simulink model "L400_airframe"  (R2024b)
settings: Solver=FixedStepAuto  StartTime=0  StopTime=20  FixedStep=5/1000  RelTol=1e-3
model workspace (MAT data in the model file):
  Sig : Simulink.Signal (value not decoded)
  Sig1 : Simulink.Signal (value not decoded)
  Sig2 : Simulink.Signal (value not decoded)
  Sig3 : Simulink.Signal (value not decoded)
  Sig4 : Simulink.Signal (value not decoded)
  Sig5 : Simulink.Signal (value not decoded)
  Sig6 : Simulink.Signal (value not decoded)
undefined symbols (not defined in the file or in its folder): convertTo, datetime, db, Earth, F, lambda, Light, MIL, WGS84, WMM2020
libraries: aerolibconvert2 x18, aerolibasang x5, aerolibtransform2 x3, aerolibwind2 x3, aerolibactuator x2, matrix_library x2, shared6dof x1, aerolibatmos2 x1, aerolibgravity2 x1
(part 3 of 4)

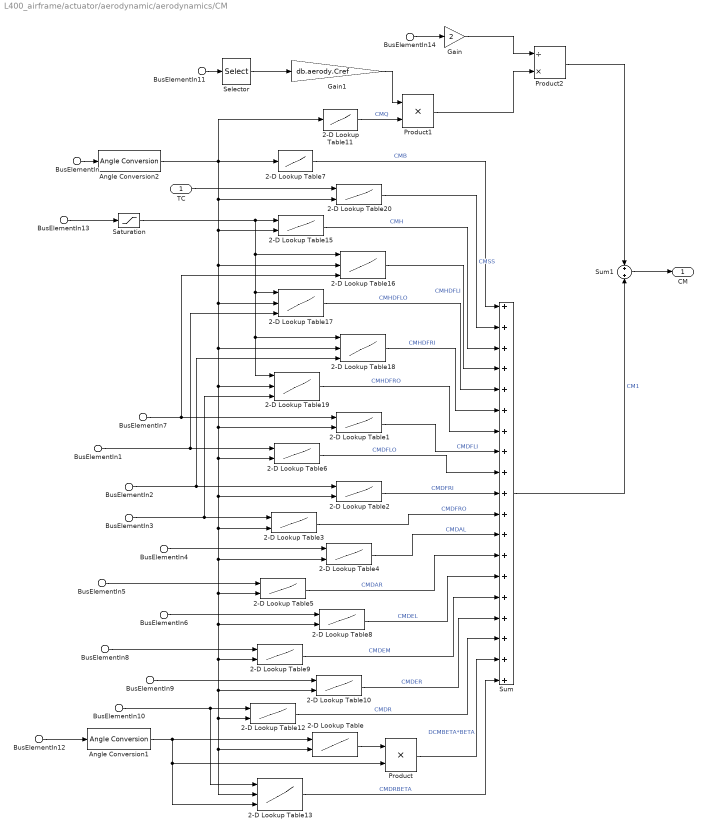
== system L400_airframe/actuator/aerodynamic/aerodynamics/CM ==
  TC : Inport
  BusElementIn7 : Inport  Port=2  PortName=surface  Element=DFLI
  BusElementIn1 : Inport  Port=2  PortName=surface  Element=DFLO
  BusElementIn2 : Inport  Port=2  PortName=surface  Element=DFRI
  BusElementIn3 : Inport  Port=2  PortName=surface  Element=DFRO
  BusElementIn4 : Inport  Port=2  PortName=surface  Element=DAL
  BusElementIn5 : Inport  Port=2  PortName=surface  Element=DAR
  BusElementIn6 : Inport  Port=2  PortName=surface  Element=DEL
  BusElementIn8 : Inport  Port=2  PortName=surface  Element=DEM
  BusElementIn9 : Inport  Port=2  PortName=surface  Element=DER
  BusElementIn10 : Inport  Port=2  PortName=surface  Element=DR
  BusElementIn : Inport  Port=3  PortName=state  Element=aircraft.airdata.alpha
  BusElementIn12 : Inport  Port=3  PortName=state  Element=aircraft.airdata.beta
  BusElementIn14 : Inport  Port=3  PortName=state  Element=aircraft.airdata.airspeed
  BusElementIn13 : Inport  Port=3  PortName=state  Element=aircraft.position.agl
  BusElementIn11 : Inport  Port=3  PortName=state  Element=aircraft.attitude.p_q_r
  2-D Lookup Table : Lookup_n-D  LookupTableObject=''  BreakpointsForDimension1=db.aerody.VBETA  BreakpointsForDimension2=db.aerody.VALPHA  BreakpointsForDimension1FirstPoint=10  BreakpointsForDimension2FirstPoint=10  BreakpointsForDimension1Spacing=12  BreakpointsForDimension2Spacing=12  IndexSearchMethod=Linear search  BeginIndexSearchUsingPreviousIndexResult=on  Table=db.aerody.DCMBETA  ExtrapMethod=Clip  DiagnosticForOutOfRangeInput=Warning  InternalRulePriority=Speed  RndMeth=Simplest
      settings: InputPortMap=u0,u1
  2-D Lookup Table1 : Lookup_n-D  LookupTableObject=''  BreakpointsForDimension1=db.aerody.VDF  BreakpointsForDimension2=db.aerody.VALPHA  BreakpointsForDimension1FirstPoint=10  BreakpointsForDimension2FirstPoint=10  BreakpointsForDimension1Spacing=12  BreakpointsForDimension2Spacing=12  IndexSearchMethod=Linear search  BeginIndexSearchUsingPreviousIndexResult=on  Table=db.aerody.CMDFLI  ExtrapMethod=Clip  DiagnosticForOutOfRangeInput=Warning  InternalRulePriority=Speed  RndMeth=Simplest
      settings: InputPortMap=u0,u1
  2-D Lookup Table10 : Lookup_n-D  LookupTableObject=''  BreakpointsForDimension1=db.aerody.VDE  BreakpointsForDimension2=db.aerody.VALPHA  BreakpointsForDimension1FirstPoint=10  BreakpointsForDimension2FirstPoint=10  BreakpointsForDimension1Spacing=12  BreakpointsForDimension2Spacing=12  IndexSearchMethod=Linear search  BeginIndexSearchUsingPreviousIndexResult=on  Table=db.aerody.CMDER  ExtrapMethod=Clip  DiagnosticForOutOfRangeInput=Warning  InternalRulePriority=Speed  RndMeth=Simplest
      settings: InputPortMap=u0,u1
  2-D Lookup Table11 : Lookup_n-D  NumberOfTableDimensions=1  LookupTableObject=''  BreakpointsForDimension1=db.aerody.VALPHA  BreakpointsForDimension2=aerody.basic.cx.beta  BreakpointsForDimension1FirstPoint=10  BreakpointsForDimension2FirstPoint=10  BreakpointsForDimension1Spacing=12  BreakpointsForDimension2Spacing=12  IndexSearchMethod=Linear search  BeginIndexSearchUsingPreviousIndexResult=on  Table=db.dds.CMQ  ExtrapMethod=Clip  DiagnosticForOutOfRangeInput=Warning  InternalRulePriority=Speed  RndMeth=Simplest
  2-D Lookup Table12 : Lookup_n-D  LookupTableObject=''  BreakpointsForDimension1=db.aerody.VDR  BreakpointsForDimension2=db.aerody.VALPHA  BreakpointsForDimension1FirstPoint=10  BreakpointsForDimension2FirstPoint=10  BreakpointsForDimension1Spacing=12  BreakpointsForDimension2Spacing=12  IndexSearchMethod=Linear search  BeginIndexSearchUsingPreviousIndexResult=on  Table=db.aerody.CMDR  ExtrapMethod=Clip  DiagnosticForOutOfRangeInput=Warning  InternalRulePriority=Speed  RndMeth=Simplest
      settings: InputPortMap=u0,u1
  2-D Lookup Table13 : Lookup_n-D  NumberOfTableDimensions=3  LookupTableObject=''  BreakpointsForDimension1=db.aerody.VDR  BreakpointsForDimension2=db.aerody.VALPHA  BreakpointsForDimension3=db.aerody.VBETA  BreakpointsForDimension1FirstPoint=10  BreakpointsForDimension2FirstPoint=10  BreakpointsForDimension1Spacing=12  BreakpointsForDimension2Spacing=12  IndexSearchMethod=Linear search  BeginIndexSearchUsingPreviousIndexResult=on  Table=db.aerody.CMDRBETA  ExtrapMethod=Clip  DiagnosticForOutOfRangeInput=Warning  InternalRulePriority=Speed  RndMeth=Simplest
      settings: InputPortMap=u0,u1,u2
  2-D Lookup Table15 : Lookup_n-D  LookupTableObject=''  BreakpointsForDimension1=db.aerody.VH  BreakpointsForDimension2=db.aerody.VALPHA  BreakpointsForDimension1FirstPoint=10  BreakpointsForDimension2FirstPoint=10  BreakpointsForDimension1Spacing=12  BreakpointsForDimension2Spacing=12  IndexSearchMethod=Linear search  BeginIndexSearchUsingPreviousIndexResult=on  Table=db.aerody.CMH  ExtrapMethod=Clip  DiagnosticForOutOfRangeInput=Warning  InternalRulePriority=Speed  RndMeth=Simplest
      settings: InputPortMap=u0,u1
  2-D Lookup Table16 : Lookup_n-D  NumberOfTableDimensions=3  LookupTableObject=''  BreakpointsForDimension1=db.aerody.VH  BreakpointsForDimension2=db.aerody.VALPHA  BreakpointsForDimension3=db.aerody.VDF  BreakpointsForDimension1FirstPoint=10  BreakpointsForDimension2FirstPoint=10  BreakpointsForDimension1Spacing=12  BreakpointsForDimension2Spacing=12  IndexSearchMethod=Linear search  BeginIndexSearchUsingPreviousIndexResult=on  Table=db.aerody.CMHDFLI  ExtrapMethod=Clip  DiagnosticForOutOfRangeInput=Warning  InternalRulePriority=Speed  RndMeth=Simplest
      settings: InputPortMap=u0,u1,u2
  2-D Lookup Table17 : Lookup_n-D  NumberOfTableDimensions=3  LookupTableObject=''  BreakpointsForDimension1=db.aerody.VH  BreakpointsForDimension2=db.aerody.VALPHA  BreakpointsForDimension3=db.aerody.VDF  BreakpointsForDimension1FirstPoint=10  BreakpointsForDimension2FirstPoint=10  BreakpointsForDimension1Spacing=12  BreakpointsForDimension2Spacing=12  IndexSearchMethod=Linear search  BeginIndexSearchUsingPreviousIndexResult=on  Table=db.aerody.CMHDFLO  ExtrapMethod=Clip  DiagnosticForOutOfRangeInput=Warning  InternalRulePriority=Speed  RndMeth=Simplest
      settings: InputPortMap=u0,u1,u2
  2-D Lookup Table18 : Lookup_n-D  NumberOfTableDimensions=3  LookupTableObject=''  BreakpointsForDimension1=db.aerody.VH  BreakpointsForDimension2=db.aerody.VALPHA  BreakpointsForDimension3=db.aerody.VDF  BreakpointsForDimension1FirstPoint=10  BreakpointsForDimension2FirstPoint=10  BreakpointsForDimension1Spacing=12  BreakpointsForDimension2Spacing=12  IndexSearchMethod=Linear search  BeginIndexSearchUsingPreviousIndexResult=on  Table=db.aerody.CMHDFRI  ExtrapMethod=Clip  DiagnosticForOutOfRangeInput=Warning  InternalRulePriority=Speed  RndMeth=Simplest
      settings: InputPortMap=u0,u1,u2
  2-D Lookup Table19 : Lookup_n-D  NumberOfTableDimensions=3  LookupTableObject=''  BreakpointsForDimension1=db.aerody.VH  BreakpointsForDimension2=db.aerody.VALPHA  BreakpointsForDimension3=db.aerody.VDF  BreakpointsForDimension1FirstPoint=10  BreakpointsForDimension2FirstPoint=10  BreakpointsForDimension1Spacing=12  BreakpointsForDimension2Spacing=12  IndexSearchMethod=Linear search  BeginIndexSearchUsingPreviousIndexResult=on  Table=db.aerody.CMHDFRO  ExtrapMethod=Clip  DiagnosticForOutOfRangeInput=Warning  InternalRulePriority=Speed  RndMeth=Simplest
      settings: InputPortMap=u0,u1,u2
  2-D Lookup Table2 : Lookup_n-D  LookupTableObject=''  BreakpointsForDimension1=db.aerody.VDF  BreakpointsForDimension2=db.aerody.VALPHA  BreakpointsForDimension1FirstPoint=10  BreakpointsForDimension2FirstPoint=10  BreakpointsForDimension1Spacing=12  BreakpointsForDimension2Spacing=12  IndexSearchMethod=Linear search  BeginIndexSearchUsingPreviousIndexResult=on  Table=db.aerody.CMDFRI  ExtrapMethod=Clip  DiagnosticForOutOfRangeInput=Warning  InternalRulePriority=Speed  RndMeth=Simplest
      settings: InputPortMap=u0,u1
  2-D Lookup Table20 : Lookup_n-D  LookupTableObject=''  BreakpointsForDimension1=db.aerody.VTC  BreakpointsForDimension2=db.aerody.VALPHA  BreakpointsForDimension1FirstPoint=10  BreakpointsForDimension2FirstPoint=10  BreakpointsForDimension1Spacing=12  BreakpointsForDimension2Spacing=12  IndexSearchMethod=Linear search  BeginIndexSearchUsingPreviousIndexResult=on  Table=db.aerody.CMSS  ExtrapMethod=Clip  DiagnosticForOutOfRangeInput=Warning  InternalRulePriority=Speed  RndMeth=Simplest
      settings: InputPortMap=u0,u1
  2-D Lookup Table3 : Lookup_n-D  LookupTableObject=''  BreakpointsForDimension1=db.aerody.VDF  BreakpointsForDimension2=db.aerody.VALPHA  BreakpointsForDimension1FirstPoint=10  BreakpointsForDimension2FirstPoint=10  BreakpointsForDimension1Spacing=12  BreakpointsForDimension2Spacing=12  IndexSearchMethod=Linear search  BeginIndexSearchUsingPreviousIndexResult=on  Table=db.aerody.CMDFRO  ExtrapMethod=Clip  DiagnosticForOutOfRangeInput=Warning  InternalRulePriority=Speed  RndMeth=Simplest
      settings: InputPortMap=u0,u1
  2-D Lookup Table4 : Lookup_n-D  LookupTableObject=''  BreakpointsForDimension1=db.aerody.VDA  BreakpointsForDimension2=db.aerody.VALPHA  BreakpointsForDimension1FirstPoint=10  BreakpointsForDimension2FirstPoint=10  BreakpointsForDimension1Spacing=12  BreakpointsForDimension2Spacing=12  IndexSearchMethod=Linear search  BeginIndexSearchUsingPreviousIndexResult=on  Table=db.aerody.CMDAL  ExtrapMethod=Clip  DiagnosticForOutOfRangeInput=Warning  InternalRulePriority=Speed  RndMeth=Simplest
      settings: InputPortMap=u0,u1
  2-D Lookup Table5 : Lookup_n-D  LookupTableObject=''  BreakpointsForDimension1=db.aerody.VDA  BreakpointsForDimension2=db.aerody.VALPHA  BreakpointsForDimension1FirstPoint=10  BreakpointsForDimension2FirstPoint=10  BreakpointsForDimension1Spacing=12  BreakpointsForDimension2Spacing=12  IndexSearchMethod=Linear search  BeginIndexSearchUsingPreviousIndexResult=on  Table=db.aerody.CMDAR  ExtrapMethod=Clip  DiagnosticForOutOfRangeInput=Warning  InternalRulePriority=Speed  RndMeth=Simplest
      settings: InputPortMap=u0,u1
  2-D Lookup Table6 : Lookup_n-D  LookupTableObject=''  BreakpointsForDimension1=db.aerody.VDF  BreakpointsForDimension2=db.aerody.VALPHA  BreakpointsForDimension1FirstPoint=10  BreakpointsForDimension2FirstPoint=10  BreakpointsForDimension1Spacing=12  BreakpointsForDimension2Spacing=12  IndexSearchMethod=Linear search  BeginIndexSearchUsingPreviousIndexResult=on  Table=db.aerody.CMDFLO  ExtrapMethod=Clip  DiagnosticForOutOfRangeInput=Warning  InternalRulePriority=Speed  RndMeth=Simplest
      settings: InputPortMap=u0,u1
  2-D Lookup Table7 : Lookup_n-D  NumberOfTableDimensions=1  LookupTableObject=''  BreakpointsForDimension1=db.aerody.VALPHA  BreakpointsForDimension2=aerody.basic.cx.beta  BreakpointsForDimension1FirstPoint=10  BreakpointsForDimension2FirstPoint=10  BreakpointsForDimension1Spacing=12  BreakpointsForDimension2Spacing=12  IndexSearchMethod=Linear search  BeginIndexSearchUsingPreviousIndexResult=on  Table=db.aerody.CMB  ExtrapMethod=Clip  DiagnosticForOutOfRangeInput=Warning  InternalRulePriority=Speed  RndMeth=Simplest
  2-D Lookup Table8 : Lookup_n-D  LookupTableObject=''  BreakpointsForDimension1=db.aerody.VDE  BreakpointsForDimension2=db.aerody.VALPHA  BreakpointsForDimension1FirstPoint=10  BreakpointsForDimension2FirstPoint=10  BreakpointsForDimension1Spacing=12  BreakpointsForDimension2Spacing=12  IndexSearchMethod=Linear search  BeginIndexSearchUsingPreviousIndexResult=on  Table=db.aerody.CMDEL  ExtrapMethod=Clip  DiagnosticForOutOfRangeInput=Warning  InternalRulePriority=Speed  RndMeth=Simplest
      settings: InputPortMap=u0,u1
  2-D Lookup Table9 : Lookup_n-D  LookupTableObject=''  BreakpointsForDimension1=db.aerody.VDE  BreakpointsForDimension2=db.aerody.VALPHA  BreakpointsForDimension1FirstPoint=10  BreakpointsForDimension2FirstPoint=10  BreakpointsForDimension1Spacing=12  BreakpointsForDimension2Spacing=12  IndexSearchMethod=Linear search  BeginIndexSearchUsingPreviousIndexResult=on  Table=db.aerody.CMDEM  ExtrapMethod=Clip  DiagnosticForOutOfRangeInput=Warning  InternalRulePriority=Speed  RndMeth=Simplest
      settings: InputPortMap=u0,u1
  Angle Conversion1 : aerolibconvert2/Angle Conversion  IU=rad  OU=deg
  Angle Conversion2 : aerolibconvert2/Angle Conversion  IU=rad  OU=deg
  Gain : Gain  Gain=2
  Gain1 : Gain  Gain=db.aerody.Cref
  Product : Product
  Product1 : Product
  Product2 : Product  Inputs=/*
  Saturation : Saturate  UpperLimit=5.8  LowerLimit=0
  Selector : Selector  InputPortWidth=3  IndexOptions=Index vector (dialog)  Indices=2  OutputSizes=1
  Sum : Sum  Inputs=19
  Sum1 : Sum  Inputs=+|+
  CM : Outport
  wires:
  Sum/1 -> Sum1/2  "CM1"
  BusElementIn7/1 -> 2-D Lookup Table16/3, 2-D Lookup Table1/1
  BusElementIn1/1 -> 2-D Lookup Table17/3, 2-D Lookup Table6/1
  BusElementIn2/1 -> 2-D Lookup Table18/3, 2-D Lookup Table2/1
  BusElementIn3/1 -> 2-D Lookup Table19/3, 2-D Lookup Table3/1
  BusElementIn4/1 -> 2-D Lookup Table4/1
  BusElementIn5/1 -> 2-D Lookup Table5/1
  BusElementIn6/1 -> 2-D Lookup Table8/1
  BusElementIn8/1 -> 2-D Lookup Table9/1
  BusElementIn9/1 -> 2-D Lookup Table10/1
  BusElementIn10/1 -> 2-D Lookup Table13/1, 2-D Lookup Table12/1
  BusElementIn12/1 -> Angle Conversion1/1
  2-D Lookup Table/1 -> Product/1
  BusElementIn13/1 -> Saturation/1
  TC/1 -> 2-D Lookup Table20/1
  BusElementIn/1 -> Angle Conversion2/1
  2-D Lookup Table2/1 -> Sum/10  "CMDFRI"
  2-D Lookup Table1/1 -> Sum/8  "CMDFLI"
  2-D Lookup Table4/1 -> Sum/12  "CMDAL"
  2-D Lookup Table18/1 -> Sum/6  "CMHDFRI"
  2-D Lookup Table6/1 -> Sum/9  "CMDFLO"
  2-D Lookup Table3/1 -> Sum/11  "CMDFRO"
  2-D Lookup Table8/1 -> Sum/14  "CMDEL"
  Product/1 -> Sum/18  "DCMBETA*BETA"
  2-D Lookup Table16/1 -> Sum/4  "CMHDFLI"
  2-D Lookup Table19/1 -> Sum/7  "CMHDFRO"
  2-D Lookup Table10/1 -> Sum/16  "CMDER"
  2-D Lookup Table5/1 -> Sum/13  "CMDAR"
  2-D Lookup Table20/1 -> Sum/2  "CMSS"
  2-D Lookup Table17/1 -> Sum/5  "CMHDFLO"
  2-D Lookup Table9/1 -> Sum/15  "CMDEM"
  2-D Lookup Table15/1 -> Sum/3  "CMH"
  2-D Lookup Table12/1 -> Sum/17  "CMDR"
  2-D Lookup Table7/1 -> Sum/1  "CMB"
  2-D Lookup Table13/1 -> Sum/19  "CMDRBETA"
  BusElementIn14/1 -> Gain/1
  BusElementIn11/1 -> Selector/1
  2-D Lookup Table11/1 -> Product1/2  "CMQ"
  Gain1/1 -> Product1/1
  Gain/1 -> Product2/1
  Product1/1 -> Product2/2
  Product2/1 -> Sum1/1
  Sum1/1 -> CM/1
  Angle Conversion1/1 -> 2-D Lookup Table13/3, Product/2, 2-D Lookup Table/1
  Angle Conversion2/1 -> 2-D Lookup Table11/1, 2-D Lookup Table12/2, 2-D Lookup Table13/2, 2-D Lookup Table/2, 2-D Lookup Table10/2, 2-D Lookup Table9/2, 2-D Lookup Table8/2, 2-D Lookup Table5/2, 2-D Lookup Table4/2, 2-D Lookup Table3/2, 2-D Lookup Table2/2, 2-D Lookup Table6/2, 2-D Lookup Table1/2, 2-D Lookup Table19/2, 2-D Lookup Table18/2, 2-D Lookup Table17/2, 2-D Lookup Table16/2, 2-D Lookup Table15/2, 2-D Lookup Table20/2, 2-D Lookup Table7/1
  Selector/1 -> Gain1/1
  Saturation/1 -> 2-D Lookup Table19/1, 2-D Lookup Table18/1, 2-D Lookup Table17/1, 2-D Lookup Table16/1, 2-D Lookup Table15/1

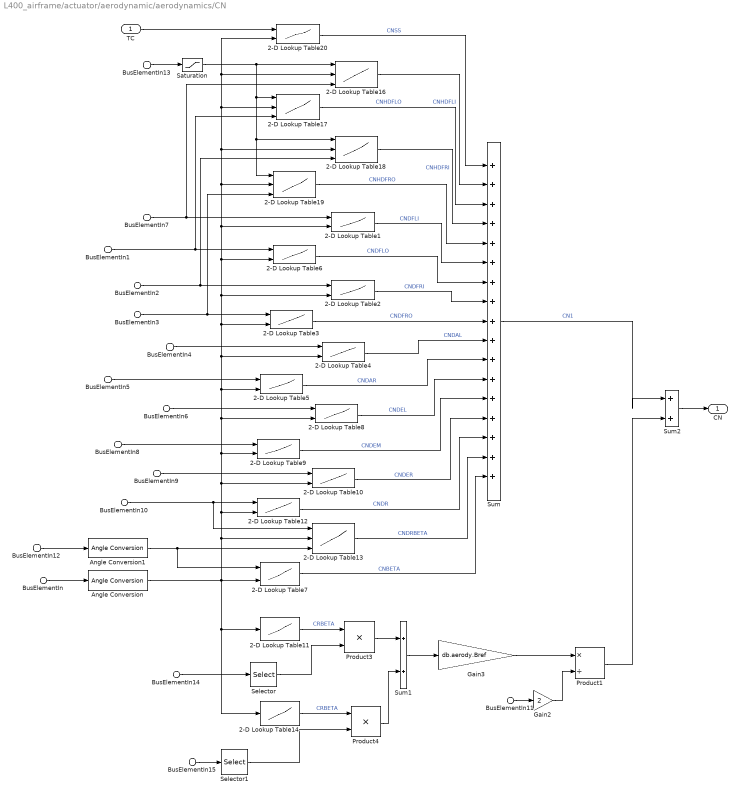
== system L400_airframe/actuator/aerodynamic/aerodynamics/CN ==
  TC : Inport
  BusElementIn7 : Inport  Port=2  PortName=surface  Element=DFLI
  BusElementIn1 : Inport  Port=2  PortName=surface  Element=DFLO
  BusElementIn2 : Inport  Port=2  PortName=surface  Element=DFRI
  BusElementIn3 : Inport  Port=2  PortName=surface  Element=DFRO
  BusElementIn4 : Inport  Port=2  PortName=surface  Element=DAL
  BusElementIn5 : Inport  Port=2  PortName=surface  Element=DAR
  BusElementIn6 : Inport  Port=2  PortName=surface  Element=DEL
  BusElementIn8 : Inport  Port=2  PortName=surface  Element=DEM
  BusElementIn9 : Inport  Port=2  PortName=surface  Element=DER
  BusElementIn10 : Inport  Port=2  PortName=surface  Element=DR
  BusElementIn : Inport  Port=3  PortName=state  Element=aircraft.airdata.alpha
  BusElementIn12 : Inport  Port=3  PortName=state  Element=aircraft.airdata.beta
  BusElementIn11 : Inport  Port=3  PortName=state  Element=aircraft.airdata.airspeed
  BusElementIn13 : Inport  Port=3  PortName=state  Element=aircraft.position.agl
  BusElementIn14 : Inport  Port=3  PortName=state  Element=aircraft.attitude.p_q_r
  BusElementIn15 : Inport  Port=3  PortName=state  Element=aircraft.attitude.p_q_r
  2-D Lookup Table1 : Lookup_n-D  LookupTableObject=''  BreakpointsForDimension1=db.aerody.VDF  BreakpointsForDimension2=db.aerody.VALPHA  BreakpointsForDimension1FirstPoint=10  BreakpointsForDimension2FirstPoint=10  BreakpointsForDimension1Spacing=12  BreakpointsForDimension2Spacing=12  IndexSearchMethod=Linear search  BeginIndexSearchUsingPreviousIndexResult=on  Table=db.aerody.CNDFLI  ExtrapMethod=Clip  DiagnosticForOutOfRangeInput=Warning  InternalRulePriority=Speed  RndMeth=Simplest
      settings: InputPortMap=u0,u1
  2-D Lookup Table10 : Lookup_n-D  LookupTableObject=''  BreakpointsForDimension1=db.aerody.VDE  BreakpointsForDimension2=db.aerody.VALPHA  BreakpointsForDimension1FirstPoint=10  BreakpointsForDimension2FirstPoint=10  BreakpointsForDimension1Spacing=12  BreakpointsForDimension2Spacing=12  IndexSearchMethod=Linear search  BeginIndexSearchUsingPreviousIndexResult=on  Table=db.aerody.CNDER  ExtrapMethod=Clip  DiagnosticForOutOfRangeInput=Warning  InternalRulePriority=Speed  RndMeth=Simplest
      settings: InputPortMap=u0,u1
  2-D Lookup Table11 : Lookup_n-D  NumberOfTableDimensions=1  LookupTableObject=''  BreakpointsForDimension1=db.dds.VALPHA  BreakpointsForDimension2=db.aerody.VALPHA  BreakpointsForDimension1FirstPoint=10  BreakpointsForDimension2FirstPoint=10  BreakpointsForDimension1Spacing=12  BreakpointsForDimension2Spacing=12  IndexSearchMethod=Linear search  BeginIndexSearchUsingPreviousIndexResult=on  Table=db.dds.CNP  ExtrapMethod=Clip  DiagnosticForOutOfRangeInput=Warning  InternalRulePriority=Speed  RndMeth=Simplest
  2-D Lookup Table12 : Lookup_n-D  LookupTableObject=''  BreakpointsForDimension1=db.aerody.VDR  BreakpointsForDimension2=db.aerody.VALPHA  BreakpointsForDimension1FirstPoint=10  BreakpointsForDimension2FirstPoint=10  BreakpointsForDimension1Spacing=12  BreakpointsForDimension2Spacing=12  IndexSearchMethod=Linear search  BeginIndexSearchUsingPreviousIndexResult=on  Table=db.aerody.CNDR  ExtrapMethod=Clip  DiagnosticForOutOfRangeInput=Warning  InternalRulePriority=Speed  RndMeth=Simplest
      settings: InputPortMap=u0,u1
  2-D Lookup Table13 : Lookup_n-D  NumberOfTableDimensions=3  LookupTableObject=''  BreakpointsForDimension1=db.aerody.VDR  BreakpointsForDimension2=db.aerody.VALPHA  BreakpointsForDimension3=db.aerody.VBETA  BreakpointsForDimension1FirstPoint=10  BreakpointsForDimension2FirstPoint=10  BreakpointsForDimension1Spacing=12  BreakpointsForDimension2Spacing=12  IndexSearchMethod=Linear search  BeginIndexSearchUsingPreviousIndexResult=on  Table=db.aerody.CNDRBETA  ExtrapMethod=Clip  DiagnosticForOutOfRangeInput=Warning  InternalRulePriority=Speed  RndMeth=Simplest
      settings: InputPortMap=u0,u1,u2
  2-D Lookup Table14 : Lookup_n-D  NumberOfTableDimensions=1  LookupTableObject=''  BreakpointsForDimension1=db.dds.VALPHA  BreakpointsForDimension2=db.aerody.VALPHA  BreakpointsForDimension1FirstPoint=10  BreakpointsForDimension2FirstPoint=10  BreakpointsForDimension1Spacing=12  BreakpointsForDimension2Spacing=12  IndexSearchMethod=Linear search  BeginIndexSearchUsingPreviousIndexResult=on  Table=db.dds.CRR  ExtrapMethod=Clip  DiagnosticForOutOfRangeInput=Warning  InternalRulePriority=Speed  RndMeth=Simplest
  2-D Lookup Table16 : Lookup_n-D  NumberOfTableDimensions=3  LookupTableObject=''  BreakpointsForDimension1=db.aerody.VH  BreakpointsForDimension2=db.aerody.VALPHA  BreakpointsForDimension3=db.aerody.VDF  BreakpointsForDimension1FirstPoint=10  BreakpointsForDimension2FirstPoint=10  BreakpointsForDimension1Spacing=12  BreakpointsForDimension2Spacing=12  IndexSearchMethod=Linear search  BeginIndexSearchUsingPreviousIndexResult=on  Table=db.aerody.CNHDFLI  ExtrapMethod=Clip  DiagnosticForOutOfRangeInput=Warning  InternalRulePriority=Speed  RndMeth=Simplest
      settings: InputPortMap=u0,u1,u2
  2-D Lookup Table17 : Lookup_n-D  NumberOfTableDimensions=3  LookupTableObject=''  BreakpointsForDimension1=db.aerody.VH  BreakpointsForDimension2=db.aerody.VALPHA  BreakpointsForDimension3=db.aerody.VDF  BreakpointsForDimension1FirstPoint=10  BreakpointsForDimension2FirstPoint=10  BreakpointsForDimension1Spacing=12  BreakpointsForDimension2Spacing=12  IndexSearchMethod=Linear search  BeginIndexSearchUsingPreviousIndexResult=on  Table=db.aerody.CNHDFLO  ExtrapMethod=Clip  DiagnosticForOutOfRangeInput=Warning  InternalRulePriority=Speed  RndMeth=Simplest
      settings: InputPortMap=u0,u1,u2
  2-D Lookup Table18 : Lookup_n-D  NumberOfTableDimensions=3  LookupTableObject=''  BreakpointsForDimension1=db.aerody.VH  BreakpointsForDimension2=db.aerody.VALPHA  BreakpointsForDimension3=db.aerody.VDF  BreakpointsForDimension1FirstPoint=10  BreakpointsForDimension2FirstPoint=10  BreakpointsForDimension1Spacing=12  BreakpointsForDimension2Spacing=12  IndexSearchMethod=Linear search  BeginIndexSearchUsingPreviousIndexResult=on  Table=db.aerody.CNHDFRI  ExtrapMethod=Clip  DiagnosticForOutOfRangeInput=Warning  InternalRulePriority=Speed  RndMeth=Simplest
      settings: InputPortMap=u0,u1,u2
  2-D Lookup Table19 : Lookup_n-D  NumberOfTableDimensions=3  LookupTableObject=''  BreakpointsForDimension1=db.aerody.VH  BreakpointsForDimension2=db.aerody.VALPHA  BreakpointsForDimension3=db.aerody.VDF  BreakpointsForDimension1FirstPoint=10  BreakpointsForDimension2FirstPoint=10  BreakpointsForDimension1Spacing=12  BreakpointsForDimension2Spacing=12  IndexSearchMethod=Linear search  BeginIndexSearchUsingPreviousIndexResult=on  Table=db.aerody.CNHDFRO  ExtrapMethod=Clip  DiagnosticForOutOfRangeInput=Warning  InternalRulePriority=Speed  RndMeth=Simplest
      settings: InputPortMap=u0,u1,u2
  2-D Lookup Table2 : Lookup_n-D  LookupTableObject=''  BreakpointsForDimension1=db.aerody.VDF  BreakpointsForDimension2=db.aerody.VALPHA  BreakpointsForDimension1FirstPoint=10  BreakpointsForDimension2FirstPoint=10  BreakpointsForDimension1Spacing=12  BreakpointsForDimension2Spacing=12  IndexSearchMethod=Linear search  BeginIndexSearchUsingPreviousIndexResult=on  Table=db.aerody.CNDFRI  ExtrapMethod=Clip  DiagnosticForOutOfRangeInput=Warning  InternalRulePriority=Speed  RndMeth=Simplest
      settings: InputPortMap=u0,u1
  2-D Lookup Table20 : Lookup_n-D  LookupTableObject=''  BreakpointsForDimension1=db.aerody.VTC  BreakpointsForDimension2=db.aerody.VALPHA  BreakpointsForDimension1FirstPoint=10  BreakpointsForDimension2FirstPoint=10  BreakpointsForDimension1Spacing=12  BreakpointsForDimension2Spacing=12  IndexSearchMethod=Linear search  BeginIndexSearchUsingPreviousIndexResult=on  Table=db.aerody.CNSS  ExtrapMethod=Clip  DiagnosticForOutOfRangeInput=Warning  InternalRulePriority=Speed  RndMeth=Simplest
      settings: InputPortMap=u0,u1
  2-D Lookup Table3 : Lookup_n-D  LookupTableObject=''  BreakpointsForDimension1=db.aerody.VDF  BreakpointsForDimension2=db.aerody.VALPHA  BreakpointsForDimension1FirstPoint=10  BreakpointsForDimension2FirstPoint=10  BreakpointsForDimension1Spacing=12  BreakpointsForDimension2Spacing=12  IndexSearchMethod=Linear search  BeginIndexSearchUsingPreviousIndexResult=on  Table=db.aerody.CNDFRO  ExtrapMethod=Clip  DiagnosticForOutOfRangeInput=Warning  InternalRulePriority=Speed  RndMeth=Simplest
      settings: InputPortMap=u0,u1
  2-D Lookup Table4 : Lookup_n-D  LookupTableObject=''  BreakpointsForDimension1=db.aerody.VDA  BreakpointsForDimension2=db.aerody.VALPHA  BreakpointsForDimension1FirstPoint=10  BreakpointsForDimension2FirstPoint=10  BreakpointsForDimension1Spacing=12  BreakpointsForDimension2Spacing=12  IndexSearchMethod=Linear search  BeginIndexSearchUsingPreviousIndexResult=on  Table=db.aerody.CNDAL  ExtrapMethod=Clip  DiagnosticForOutOfRangeInput=Warning  InternalRulePriority=Speed  RndMeth=Simplest
      settings: InputPortMap=u0,u1
  2-D Lookup Table5 : Lookup_n-D  LookupTableObject=''  BreakpointsForDimension1=db.aerody.VDA  BreakpointsForDimension2=db.aerody.VALPHA  BreakpointsForDimension1FirstPoint=10  BreakpointsForDimension2FirstPoint=10  BreakpointsForDimension1Spacing=12  BreakpointsForDimension2Spacing=12  IndexSearchMethod=Linear search  BeginIndexSearchUsingPreviousIndexResult=on  Table=db.aerody.CNDAR  ExtrapMethod=Clip  DiagnosticForOutOfRangeInput=Warning  InternalRulePriority=Speed  RndMeth=Simplest
      settings: InputPortMap=u0,u1
  2-D Lookup Table6 : Lookup_n-D  LookupTableObject=''  BreakpointsForDimension1=db.aerody.VDF  BreakpointsForDimension2=db.aerody.VALPHA  BreakpointsForDimension1FirstPoint=10  BreakpointsForDimension2FirstPoint=10  BreakpointsForDimension1Spacing=12  BreakpointsForDimension2Spacing=12  IndexSearchMethod=Linear search  BeginIndexSearchUsingPreviousIndexResult=on  Table=db.aerody.CNDFLO  ExtrapMethod=Clip  DiagnosticForOutOfRangeInput=Warning  InternalRulePriority=Speed  RndMeth=Simplest
      settings: InputPortMap=u0,u1
  2-D Lookup Table7 : Lookup_n-D  LookupTableObject=''  BreakpointsForDimension1=db.aerody.VBETA  BreakpointsForDimension2=db.aerody.VALPHA  BreakpointsForDimension1FirstPoint=10  BreakpointsForDimension2FirstPoint=10  BreakpointsForDimension1Spacing=12  BreakpointsForDimension2Spacing=12  IndexSearchMethod=Linear search  BeginIndexSearchUsingPreviousIndexResult=on  Table=db.aerody.CNBETA  ExtrapMethod=Clip  DiagnosticForOutOfRangeInput=Warning  InternalRulePriority=Speed  RndMeth=Simplest
      settings: InputPortMap=u0,u1
  2-D Lookup Table8 : Lookup_n-D  LookupTableObject=''  BreakpointsForDimension1=db.aerody.VDE  BreakpointsForDimension2=db.aerody.VALPHA  BreakpointsForDimension1FirstPoint=10  BreakpointsForDimension2FirstPoint=10  BreakpointsForDimension1Spacing=12  BreakpointsForDimension2Spacing=12  IndexSearchMethod=Linear search  BeginIndexSearchUsingPreviousIndexResult=on  Table=db.aerody.CNDEL  ExtrapMethod=Clip  DiagnosticForOutOfRangeInput=Warning  InternalRulePriority=Speed  RndMeth=Simplest
      settings: InputPortMap=u0,u1
  2-D Lookup Table9 : Lookup_n-D  LookupTableObject=''  BreakpointsForDimension1=db.aerody.VDE  BreakpointsForDimension2=db.aerody.VALPHA  BreakpointsForDimension1FirstPoint=10  BreakpointsForDimension2FirstPoint=10  BreakpointsForDimension1Spacing=12  BreakpointsForDimension2Spacing=12  IndexSearchMethod=Linear search  BeginIndexSearchUsingPreviousIndexResult=on  Table=db.aerody.CNDEM  ExtrapMethod=Clip  DiagnosticForOutOfRangeInput=Warning  InternalRulePriority=Speed  RndMeth=Simplest
      settings: InputPortMap=u0,u1
  Angle Conversion : aerolibconvert2/Angle Conversion  IU=rad  OU=deg
  Angle Conversion1 : aerolibconvert2/Angle Conversion  IU=rad  OU=deg
  Gain2 : Gain  Gain=2
  Gain3 : Gain  Gain=db.aerody.Bref
  Product1 : Product  Inputs=*/
  Product3 : Product  Inputs=**
  Product4 : Product  Inputs=**
  Saturation : Saturate  UpperLimit=5.8  LowerLimit=0
  Selector : Selector  InputPortWidth=3  IndexOptions=Index vector (dialog)  Indices=1  OutputSizes=1
  Selector1 : Selector  InputPortWidth=3  IndexOptions=Index vector (dialog)  Indices=3  OutputSizes=1
  Sum : Sum  Inputs=17
  Sum1 : Sum  Inputs=2
  Sum2 : Sum  Inputs=|++
  CN : Outport
  wires:
  BusElementIn12/1 -> Angle Conversion1/1
  Sum/1 -> Sum2/1  "CN1"
  BusElementIn7/1 -> 2-D Lookup Table16/3, 2-D Lookup Table1/1
  BusElementIn1/1 -> 2-D Lookup Table17/3, 2-D Lookup Table6/1
  BusElementIn2/1 -> 2-D Lookup Table18/3, 2-D Lookup Table2/1
  BusElementIn3/1 -> 2-D Lookup Table19/3, 2-D Lookup Table3/1
  BusElementIn4/1 -> 2-D Lookup Table4/1
  BusElementIn5/1 -> 2-D Lookup Table5/1
  BusElementIn6/1 -> 2-D Lookup Table8/1
  BusElementIn8/1 -> 2-D Lookup Table9/1
  BusElementIn9/1 -> 2-D Lookup Table10/1
  BusElementIn10/1 -> 2-D Lookup Table13/1, 2-D Lookup Table12/1
  BusElementIn13/1 -> Saturation/1
  TC/1 -> 2-D Lookup Table20/1
  BusElementIn/1 -> Angle Conversion/1
  2-D Lookup Table2/1 -> Sum/8  "CNDFRI"
  2-D Lookup Table4/1 -> Sum/10  "CNDAL"
  2-D Lookup Table1/1 -> Sum/6  "CNDFLI"
  2-D Lookup Table3/1 -> Sum/9  "CNDFRO"
  2-D Lookup Table8/1 -> Sum/12  "CNDEL"
  2-D Lookup Table18/1 -> Sum/4  "CNHDFRI"
  2-D Lookup Table6/1 -> Sum/7  "CNDFLO"
  2-D Lookup Table5/1 -> Sum/11  "CNDAR"
  2-D Lookup Table10/1 -> Sum/14  "CNDER"
  2-D Lookup Table16/1 -> Sum/2  "CNHDFLI"
  2-D Lookup Table19/1 -> Sum/5  "CNHDFRO"
  2-D Lookup Table9/1 -> Sum/13  "CNDEM"
  2-D Lookup Table13/1 -> Sum/16  "CNDRBETA"
  2-D Lookup Table17/1 -> Sum/3  "CNHDFLO"
  2-D Lookup Table12/1 -> Sum/15  "CNDR"
  2-D Lookup Table20/1 -> Sum/1  "CNSS"
  2-D Lookup Table7/1 -> Sum/17  "CNBETA"
  Sum1/1 -> Gain3/1
  BusElementIn11/1 -> Gain2/1
  Selector1/1 -> Product4/2
  Selector/1 -> Product3/2
  2-D Lookup Table11/1 -> Product3/1  "CRBETA"
  2-D Lookup Table14/1 -> Product4/1  "CRBETA"
  Product3/1 -> Sum1/1
  Product4/1 -> Sum1/2
  Product1/1 -> Sum2/2
  Sum2/1 -> CN/1
  Angle Conversion/1 -> 2-D Lookup Table14/1, 2-D Lookup Table11/1, 2-D Lookup Table20/2, 2-D Lookup Table16/2, 2-D Lookup Table17/2, 2-D Lookup Table18/2, 2-D Lookup Table19/2, 2-D Lookup Table1/2, 2-D Lookup Table6/2, 2-D Lookup Table2/2, 2-D Lookup Table3/2, 2-D Lookup Table4/2, 2-D Lookup Table5/2, 2-D Lookup Table8/2, 2-D Lookup Table9/2, 2-D Lookup Table10/2, 2-D Lookup Table12/2, 2-D Lookup Table13/2, 2-D Lookup Table7/2
  Angle Conversion1/1 -> 2-D Lookup Table7/1, 2-D Lookup Table13/3
  BusElementIn15/1 -> Selector1/1
  BusElementIn14/1 -> Selector/1
  Saturation/1 -> 2-D Lookup Table17/1, 2-D Lookup Table18/1, 2-D Lookup Table19/1, 2-D Lookup Table16/1
  Gain3/1 -> Product1/1
  Gain2/1 -> Product1/2

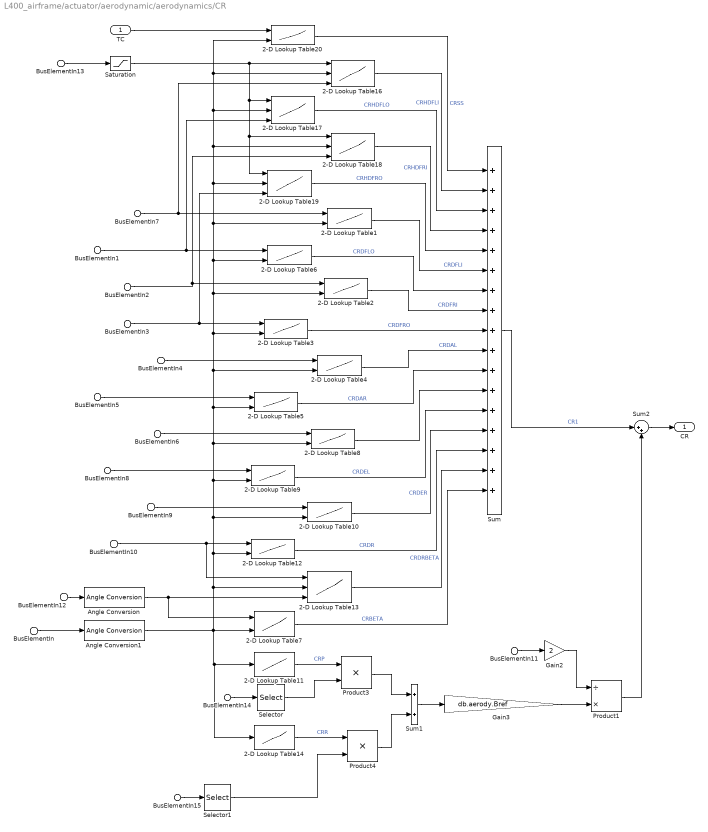
== system L400_airframe/actuator/aerodynamic/aerodynamics/CR ==
  TC : Inport
  BusElementIn7 : Inport  Port=2  PortName=surface  Element=DFLI
  BusElementIn1 : Inport  Port=2  PortName=surface  Element=DFLO
  BusElementIn2 : Inport  Port=2  PortName=surface  Element=DFRI
  BusElementIn3 : Inport  Port=2  PortName=surface  Element=DFRO
  BusElementIn4 : Inport  Port=2  PortName=surface  Element=DAL
  BusElementIn5 : Inport  Port=2  PortName=surface  Element=DAR
  BusElementIn6 : Inport  Port=2  PortName=surface  Element=DEL
  BusElementIn8 : Inport  Port=2  PortName=surface  Element=DEM
  BusElementIn9 : Inport  Port=2  PortName=surface  Element=DER
  BusElementIn10 : Inport  Port=2  PortName=surface  Element=DR
  BusElementIn : Inport  Port=3  PortName=state  Element=aircraft.airdata.alpha
  BusElementIn12 : Inport  Port=3  PortName=state  Element=aircraft.airdata.beta
  BusElementIn11 : Inport  Port=3  PortName=state  Element=aircraft.airdata.airspeed
  BusElementIn13 : Inport  Port=3  PortName=state  Element=aircraft.position.agl
  BusElementIn14 : Inport  Port=3  PortName=state  Element=aircraft.attitude.p_q_r
  BusElementIn15 : Inport  Port=3  PortName=state  Element=aircraft.attitude.p_q_r
  2-D Lookup Table1 : Lookup_n-D  LookupTableObject=''  BreakpointsForDimension1=db.aerody.VDF  BreakpointsForDimension2=db.aerody.VALPHA  BreakpointsForDimension1FirstPoint=10  BreakpointsForDimension2FirstPoint=10  BreakpointsForDimension1Spacing=12  BreakpointsForDimension2Spacing=12  IndexSearchMethod=Linear search  BeginIndexSearchUsingPreviousIndexResult=on  Table=db.aerody.CRDFLI  ExtrapMethod=Clip  DiagnosticForOutOfRangeInput=Warning  InternalRulePriority=Speed  RndMeth=Simplest
      settings: InputPortMap=u0,u1
  2-D Lookup Table10 : Lookup_n-D  LookupTableObject=''  BreakpointsForDimension1=db.aerody.VDE  BreakpointsForDimension2=db.aerody.VALPHA  BreakpointsForDimension1FirstPoint=10  BreakpointsForDimension2FirstPoint=10  BreakpointsForDimension1Spacing=12  BreakpointsForDimension2Spacing=12  IndexSearchMethod=Linear search  BeginIndexSearchUsingPreviousIndexResult=on  Table=db.aerody.CRDER  ExtrapMethod=Clip  DiagnosticForOutOfRangeInput=Warning  InternalRulePriority=Speed  RndMeth=Simplest
      settings: InputPortMap=u0,u1
  2-D Lookup Table11 : Lookup_n-D  NumberOfTableDimensions=1  LookupTableObject=''  BreakpointsForDimension1=db.dds.VALPHA  BreakpointsForDimension2=db.aerody.VALPHA  BreakpointsForDimension1FirstPoint=10  BreakpointsForDimension2FirstPoint=10  BreakpointsForDimension1Spacing=12  BreakpointsForDimension2Spacing=12  IndexSearchMethod=Linear search  BeginIndexSearchUsingPreviousIndexResult=on  Table=db.dds.CRP  ExtrapMethod=Clip  DiagnosticForOutOfRangeInput=Warning  InternalRulePriority=Speed  RndMeth=Simplest
  2-D Lookup Table12 : Lookup_n-D  LookupTableObject=''  BreakpointsForDimension1=db.aerody.VDR  BreakpointsForDimension2=db.aerody.VALPHA  BreakpointsForDimension1FirstPoint=10  BreakpointsForDimension2FirstPoint=10  BreakpointsForDimension1Spacing=12  BreakpointsForDimension2Spacing=12  IndexSearchMethod=Linear search  BeginIndexSearchUsingPreviousIndexResult=on  Table=db.aerody.CRDR  ExtrapMethod=Clip  DiagnosticForOutOfRangeInput=Warning  InternalRulePriority=Speed  RndMeth=Simplest
      settings: InputPortMap=u0,u1
  2-D Lookup Table13 : Lookup_n-D  NumberOfTableDimensions=3  LookupTableObject=''  BreakpointsForDimension1=db.aerody.VDR  BreakpointsForDimension2=db.aerody.VALPHA  BreakpointsForDimension3=db.aerody.VBETA  BreakpointsForDimension1FirstPoint=10  BreakpointsForDimension2FirstPoint=10  BreakpointsForDimension1Spacing=12  BreakpointsForDimension2Spacing=12  IndexSearchMethod=Linear search  BeginIndexSearchUsingPreviousIndexResult=on  Table=db.aerody.CRDRBETA  ExtrapMethod=Clip  DiagnosticForOutOfRangeInput=Warning  InternalRulePriority=Speed  RndMeth=Simplest
      settings: InputPortMap=u0,u1,u2
  2-D Lookup Table14 : Lookup_n-D  NumberOfTableDimensions=1  LookupTableObject=''  BreakpointsForDimension1=db.dds.VALPHA  BreakpointsForDimension2=db.aerody.VALPHA  BreakpointsForDimension1FirstPoint=10  BreakpointsForDimension2FirstPoint=10  BreakpointsForDimension1Spacing=12  BreakpointsForDimension2Spacing=12  IndexSearchMethod=Linear search  BeginIndexSearchUsingPreviousIndexResult=on  Table=db.dds.CRR  ExtrapMethod=Clip  DiagnosticForOutOfRangeInput=Warning  InternalRulePriority=Speed  RndMeth=Simplest
  2-D Lookup Table16 : Lookup_n-D  NumberOfTableDimensions=3  LookupTableObject=''  BreakpointsForDimension1=db.aerody.VH  BreakpointsForDimension2=db.aerody.VALPHA  BreakpointsForDimension3=db.aerody.VDF  BreakpointsForDimension1FirstPoint=10  BreakpointsForDimension2FirstPoint=10  BreakpointsForDimension1Spacing=12  BreakpointsForDimension2Spacing=12  IndexSearchMethod=Linear search  BeginIndexSearchUsingPreviousIndexResult=on  Table=db.aerody.CRHDFLI  ExtrapMethod=Clip  DiagnosticForOutOfRangeInput=Warning  InternalRulePriority=Speed  RndMeth=Simplest
      settings: InputPortMap=u0,u1,u2
  2-D Lookup Table17 : Lookup_n-D  NumberOfTableDimensions=3  LookupTableObject=''  BreakpointsForDimension1=db.aerody.VH  BreakpointsForDimension2=db.aerody.VALPHA  BreakpointsForDimension3=db.aerody.VDF  BreakpointsForDimension1FirstPoint=10  BreakpointsForDimension2FirstPoint=10  BreakpointsForDimension1Spacing=12  BreakpointsForDimension2Spacing=12  IndexSearchMethod=Linear search  BeginIndexSearchUsingPreviousIndexResult=on  Table=db.aerody.CRHDFLO  ExtrapMethod=Clip  DiagnosticForOutOfRangeInput=Warning  InternalRulePriority=Speed  RndMeth=Simplest
      settings: InputPortMap=u0,u1,u2
  2-D Lookup Table18 : Lookup_n-D  NumberOfTableDimensions=3  LookupTableObject=''  BreakpointsForDimension1=db.aerody.VH  BreakpointsForDimension2=db.aerody.VALPHA  BreakpointsForDimension3=db.aerody.VDF  BreakpointsForDimension1FirstPoint=10  BreakpointsForDimension2FirstPoint=10  BreakpointsForDimension1Spacing=12  BreakpointsForDimension2Spacing=12  IndexSearchMethod=Linear search  BeginIndexSearchUsingPreviousIndexResult=on  Table=db.aerody.CRHDFRI  ExtrapMethod=Clip  DiagnosticForOutOfRangeInput=Warning  InternalRulePriority=Speed  RndMeth=Simplest
      settings: InputPortMap=u0,u1,u2
  2-D Lookup Table19 : Lookup_n-D  NumberOfTableDimensions=3  LookupTableObject=''  BreakpointsForDimension1=db.aerody.VH  BreakpointsForDimension2=db.aerody.VALPHA  BreakpointsForDimension3=db.aerody.VDF  BreakpointsForDimension1FirstPoint=10  BreakpointsForDimension2FirstPoint=10  BreakpointsForDimension1Spacing=12  BreakpointsForDimension2Spacing=12  IndexSearchMethod=Linear search  BeginIndexSearchUsingPreviousIndexResult=on  Table=db.aerody.CRHDFRO  ExtrapMethod=Clip  DiagnosticForOutOfRangeInput=Warning  InternalRulePriority=Speed  RndMeth=Simplest
      settings: InputPortMap=u0,u1,u2
  2-D Lookup Table2 : Lookup_n-D  LookupTableObject=''  BreakpointsForDimension1=db.aerody.VDF  BreakpointsForDimension2=db.aerody.VALPHA  BreakpointsForDimension1FirstPoint=10  BreakpointsForDimension2FirstPoint=10  BreakpointsForDimension1Spacing=12  BreakpointsForDimension2Spacing=12  IndexSearchMethod=Linear search  BeginIndexSearchUsingPreviousIndexResult=on  Table=db.aerody.CRDFRI  ExtrapMethod=Clip  DiagnosticForOutOfRangeInput=Warning  InternalRulePriority=Speed  RndMeth=Simplest
      settings: InputPortMap=u0,u1
  2-D Lookup Table20 : Lookup_n-D  LookupTableObject=''  BreakpointsForDimension1=db.aerody.VTC  BreakpointsForDimension2=db.aerody.VALPHA  BreakpointsForDimension1FirstPoint=10  BreakpointsForDimension2FirstPoint=10  BreakpointsForDimension1Spacing=12  BreakpointsForDimension2Spacing=12  IndexSearchMethod=Linear search  BeginIndexSearchUsingPreviousIndexResult=on  Table=db.aerody.CRSS  ExtrapMethod=Clip  DiagnosticForOutOfRangeInput=Warning  InternalRulePriority=Speed  RndMeth=Simplest
      settings: InputPortMap=u0,u1
  2-D Lookup Table3 : Lookup_n-D  LookupTableObject=''  BreakpointsForDimension1=db.aerody.VDF  BreakpointsForDimension2=db.aerody.VALPHA  BreakpointsForDimension1FirstPoint=10  BreakpointsForDimension2FirstPoint=10  BreakpointsForDimension1Spacing=12  BreakpointsForDimension2Spacing=12  IndexSearchMethod=Linear search  BeginIndexSearchUsingPreviousIndexResult=on  Table=db.aerody.CRDFRO  ExtrapMethod=Clip  DiagnosticForOutOfRangeInput=Warning  InternalRulePriority=Speed  RndMeth=Simplest
      settings: InputPortMap=u0,u1
  2-D Lookup Table4 : Lookup_n-D  LookupTableObject=''  BreakpointsForDimension1=db.aerody.VDA  BreakpointsForDimension2=db.aerody.VALPHA  BreakpointsForDimension1FirstPoint=10  BreakpointsForDimension2FirstPoint=10  BreakpointsForDimension1Spacing=12  BreakpointsForDimension2Spacing=12  IndexSearchMethod=Linear search  BeginIndexSearchUsingPreviousIndexResult=on  Table=db.aerody.CRDAL  ExtrapMethod=Clip  DiagnosticForOutOfRangeInput=Warning  InternalRulePriority=Speed  RndMeth=Simplest
      settings: InputPortMap=u0,u1
  2-D Lookup Table5 : Lookup_n-D  LookupTableObject=''  BreakpointsForDimension1=db.aerody.VDA  BreakpointsForDimension2=db.aerody.VALPHA  BreakpointsForDimension1FirstPoint=10  BreakpointsForDimension2FirstPoint=10  BreakpointsForDimension1Spacing=12  BreakpointsForDimension2Spacing=12  IndexSearchMethod=Linear search  BeginIndexSearchUsingPreviousIndexResult=on  Table=db.aerody.CRDAR  ExtrapMethod=Clip  DiagnosticForOutOfRangeInput=Warning  InternalRulePriority=Speed  RndMeth=Simplest
      settings: InputPortMap=u0,u1
  2-D Lookup Table6 : Lookup_n-D  LookupTableObject=''  BreakpointsForDimension1=db.aerody.VDF  BreakpointsForDimension2=db.aerody.VALPHA  BreakpointsForDimension1FirstPoint=10  BreakpointsForDimension2FirstPoint=10  BreakpointsForDimension1Spacing=12  BreakpointsForDimension2Spacing=12  IndexSearchMethod=Linear search  BeginIndexSearchUsingPreviousIndexResult=on  Table=db.aerody.CRDFLO  ExtrapMethod=Clip  DiagnosticForOutOfRangeInput=Warning  InternalRulePriority=Speed  RndMeth=Simplest
      settings: InputPortMap=u0,u1
  2-D Lookup Table7 : Lookup_n-D  LookupTableObject=''  BreakpointsForDimension1=db.aerody.VBETA  BreakpointsForDimension2=db.aerody.VALPHA  BreakpointsForDimension1FirstPoint=10  BreakpointsForDimension2FirstPoint=10  BreakpointsForDimension1Spacing=12  BreakpointsForDimension2Spacing=12  IndexSearchMethod=Linear search  BeginIndexSearchUsingPreviousIndexResult=on  Table=db.aerody.CRBETA  ExtrapMethod=Clip  DiagnosticForOutOfRangeInput=Warning  InternalRulePriority=Speed  RndMeth=Simplest
      settings: InputPortMap=u0,u1
  2-D Lookup Table8 : Lookup_n-D  LookupTableObject=''  BreakpointsForDimension1=db.aerody.VDE  BreakpointsForDimension2=db.aerody.VALPHA  BreakpointsForDimension1FirstPoint=10  BreakpointsForDimension2FirstPoint=10  BreakpointsForDimension1Spacing=12  BreakpointsForDimension2Spacing=12  IndexSearchMethod=Linear search  BeginIndexSearchUsingPreviousIndexResult=on  Table=db.aerody.CRDEL  ExtrapMethod=Clip  DiagnosticForOutOfRangeInput=Warning  InternalRulePriority=Speed  RndMeth=Simplest
      settings: InputPortMap=u0,u1
  2-D Lookup Table9 : Lookup_n-D  LookupTableObject=''  BreakpointsForDimension1=db.aerody.VDE  BreakpointsForDimension2=db.aerody.VALPHA  BreakpointsForDimension1FirstPoint=10  BreakpointsForDimension2FirstPoint=10  BreakpointsForDimension1Spacing=12  BreakpointsForDimension2Spacing=12  IndexSearchMethod=Linear search  BeginIndexSearchUsingPreviousIndexResult=on  Table=db.aerody.CRDEM  ExtrapMethod=Clip  DiagnosticForOutOfRangeInput=Warning  InternalRulePriority=Speed  RndMeth=Simplest
      settings: InputPortMap=u0,u1
  Angle Conversion : aerolibconvert2/Angle Conversion  IU=rad  OU=deg
  Angle Conversion1 : aerolibconvert2/Angle Conversion  IU=rad  OU=deg
  Gain2 : Gain  Gain=2
  Gain3 : Gain  Gain=db.aerody.Bref
  Product1 : Product  Inputs=/*
  Product3 : Product  Inputs=**
  Product4 : Product  Inputs=**
  Saturation : Saturate  UpperLimit=5.8  LowerLimit=0
  Selector : Selector  InputPortWidth=3  IndexOptions=Index vector (dialog)  Indices=1  OutputSizes=1
  Selector1 : Selector  InputPortWidth=3  IndexOptions=Index vector (dialog)  Indices=3  OutputSizes=1
  Sum : Sum  Inputs=17
  Sum1 : Sum  Inputs=2
  Sum2 : Sum  Inputs=|++
  CR : Outport
  wires:
  BusElementIn/1 -> Angle Conversion1/1
  TC/1 -> 2-D Lookup Table20/1
  BusElementIn13/1 -> Saturation/1
  BusElementIn10/1 -> 2-D Lookup Table13/1, 2-D Lookup Table12/1
  BusElementIn9/1 -> 2-D Lookup Table10/1
  BusElementIn8/1 -> 2-D Lookup Table9/1
  BusElementIn6/1 -> 2-D Lookup Table8/1
  BusElementIn5/1 -> 2-D Lookup Table5/1
  BusElementIn4/1 -> 2-D Lookup Table4/1
  BusElementIn3/1 -> 2-D Lookup Table19/3, 2-D Lookup Table3/1
  BusElementIn2/1 -> 2-D Lookup Table18/3, 2-D Lookup Table2/1
  BusElementIn1/1 -> 2-D Lookup Table6/1, 2-D Lookup Table17/3
  BusElementIn7/1 -> 2-D Lookup Table1/1, 2-D Lookup Table16/3
  Sum/1 -> Sum2/1  "CR1"
  BusElementIn12/1 -> Angle Conversion/1
  2-D Lookup Table2/1 -> Sum/8  "CRDFRI"
  2-D Lookup Table1/1 -> Sum/6  "CRDFLI"
  2-D Lookup Table4/1 -> Sum/10  "CRDAL"
  2-D Lookup Table18/1 -> Sum/4  "CRHDFRI"
  2-D Lookup Table6/1 -> Sum/7  "CRDFLO"
  2-D Lookup Table3/1 -> Sum/9  "CRDFRO"
  2-D Lookup Table8/1 -> Sum/12
  2-D Lookup Table16/1 -> Sum/2  "CRHDFLI"
  2-D Lookup Table19/1 -> Sum/5  "CRHDFRO"
  2-D Lookup Table10/1 -> Sum/14  "CRDER"
  2-D Lookup Table5/1 -> Sum/11  "CRDAR"
  2-D Lookup Table17/1 -> Sum/3  "CRHDFLO"
  2-D Lookup Table13/1 -> Sum/16  "CRDRBETA"
  2-D Lookup Table9/1 -> Sum/13  "CRDEL"
  2-D Lookup Table20/1 -> Sum/1  "CRSS"
  2-D Lookup Table12/1 -> Sum/15  "CRDR"
  2-D Lookup Table7/1 -> Sum/17  "CRBETA"
  BusElementIn11/1 -> Gain2/1
  Gain2/1 -> Product1/1
  Gain3/1 -> Product1/2
  Sum1/1 -> Gain3/1
  2-D Lookup Table11/1 -> Product3/1  "CRP"
  2-D Lookup Table14/1 -> Product4/1  "CRR"
  Selector1/1 -> Product4/2
  Selector/1 -> Product3/2
  Product3/1 -> Sum1/1
  Product4/1 -> Sum1/2
  Product1/1 -> Sum2/2
  Sum2/1 -> CR/1
  Angle Conversion/1 -> 2-D Lookup Table7/1, 2-D Lookup Table13/3
  Angle Conversion1/1 -> 2-D Lookup Table14/1, 2-D Lookup Table11/1, 2-D Lookup Table20/2, 2-D Lookup Table16/2, 2-D Lookup Table17/2, 2-D Lookup Table18/2, 2-D Lookup Table19/2, 2-D Lookup Table1/2, 2-D Lookup Table6/2, 2-D Lookup Table2/2, 2-D Lookup Table3/2, 2-D Lookup Table4/2, 2-D Lookup Table5/2, 2-D Lookup Table8/2, 2-D Lookup Table9/2, 2-D Lookup Table10/2, 2-D Lookup Table12/2, 2-D Lookup Table13/2, 2-D Lookup Table7/2
  BusElementIn14/1 -> Selector/1
  BusElementIn15/1 -> Selector1/1
  Saturation/1 -> 2-D Lookup Table19/1, 2-D Lookup Table18/1, 2-D Lookup Table17/1, 2-D Lookup Table16/1

== system L400_airframe/actuator/aerodynamic/aerodynamics/CY ==
  TC : Inport
  BusElementIn7 : Inport  Port=2  PortName=surface  Element=DFLI
  BusElementIn1 : Inport  Port=2  PortName=surface  Element=DFLO
  BusElementIn2 : Inport  Port=2  PortName=surface  Element=DFRI
  BusElementIn3 : Inport  Port=2  PortName=surface  Element=DFRO
  BusElementIn4 : Inport  Port=2  PortName=surface  Element=DAL
  BusElementIn5 : Inport  Port=2  PortName=surface  Element=DAR
  BusElementIn6 : Inport  Port=2  PortName=surface  Element=DEL
  BusElementIn8 : Inport  Port=2  PortName=surface  Element=DEM
  BusElementIn9 : Inport  Port=2  PortName=surface  Element=DER
  BusElementIn10 : Inport  Port=2  PortName=surface  Element=DR
  BusElementIn : Inport  Port=3  PortName=state  Element=aircraft.airdata.alpha
  BusElementIn12 : Inport  Port=3  PortName=state  Element=aircraft.airdata.beta
  BusElementIn13 : Inport  Port=3  PortName=state  Element=aircraft.position.agl
  Angle Conversion : aerolibconvert2/Angle Conversion  IU=rad  OU=deg
  Angle Conversion1 : aerolibconvert2/Angle Conversion  IU=rad  OU=deg
  Subsystem : Subsystem
  CY : Outport
  wires:
  TC/1 -> Subsystem/4(TC)
  BusElementIn13/1 -> Subsystem/3(H)
  BusElementIn7/1 -> Subsystem/5(DFLI)
  BusElementIn1/1 -> Subsystem/6(DFLO)
  BusElementIn2/1 -> Subsystem/7(DFRI)
  BusElementIn3/1 -> Subsystem/8(DFRO)
  BusElementIn4/1 -> Subsystem/9(DAL)
  BusElementIn5/1 -> Subsystem/10(DAR)
  BusElementIn6/1 -> Subsystem/11(DEL)
  BusElementIn8/1 -> Subsystem/12(DEM)
  BusElementIn9/1 -> Subsystem/13(DER)
  BusElementIn10/1 -> Subsystem/14(DR)
  BusElementIn12/1 -> Angle Conversion1/1
  BusElementIn/1 -> Angle Conversion/1
  Subsystem/1(CY) -> CY/1
  Angle Conversion/1 -> Subsystem/1(alpha)
  Angle Conversion1/1 -> Subsystem/2(beta)

== system L400_airframe/actuator/aerodynamic/actuator/Variant Subsystem/Direct Through ==
  In1 : Inport
  Out1 : Outport
  wires:
  In1/1 -> Out1/1

== system L400_airframe/actuator/aerodynamic/actuator/Variant Subsystem/Linear ==
  In1 : Inport
  Linear Second-Order Actuator : aerolibactuator/Linear Second-Order Actuator  wn_fin=1  z_fin=0.3  fin_act_0=0  fin_act_vel=0
  Out1 : Outport
  wires:
  Linear Second-Order Actuator/1 -> Out1/1
  In1/1 -> Linear Second-Order Actuator/1
